simulink model "no_zerosimulink"  (R2017b)
settings: Solver=VariableStepAuto  StartTime=0.0  StopTime=10  RelTol=1e-3  EnableMultiTasking=on
undefined symbols (not defined in the file): DiscIntNeverNeededParam, rho1, rho3, rho5, rho6, sigma1, sigma2, sigma3, sigma4, sigma5, sigma6
libraries: simulink x1
settings Model: Creator=Tuo  LastModifiedBy=柏陞
settings OptimizationCC: LifeSpan=inf
settings DebuggingCC: SFUnexpectedBacktrackingDiag=warning  SFNoUnconditionalDefaultTransitionDiag=warning  SFExecutionAtInitializationDiag=none
settings CodeAppCC: StateflowObjectComments=on
settings GRTTargetCC: TargetLangStandard=C89/C90 (ANSI)  GeneratePreprocessorConditionals=Disable all
settings ConfigComp: CovMetricSettings=dw  CovHtmlReporting=on  CovSaveCumulativeToWorkspaceVar=on  CovSaveSingleToWorkspaceVar=on  CovExternalEMLEnable=off

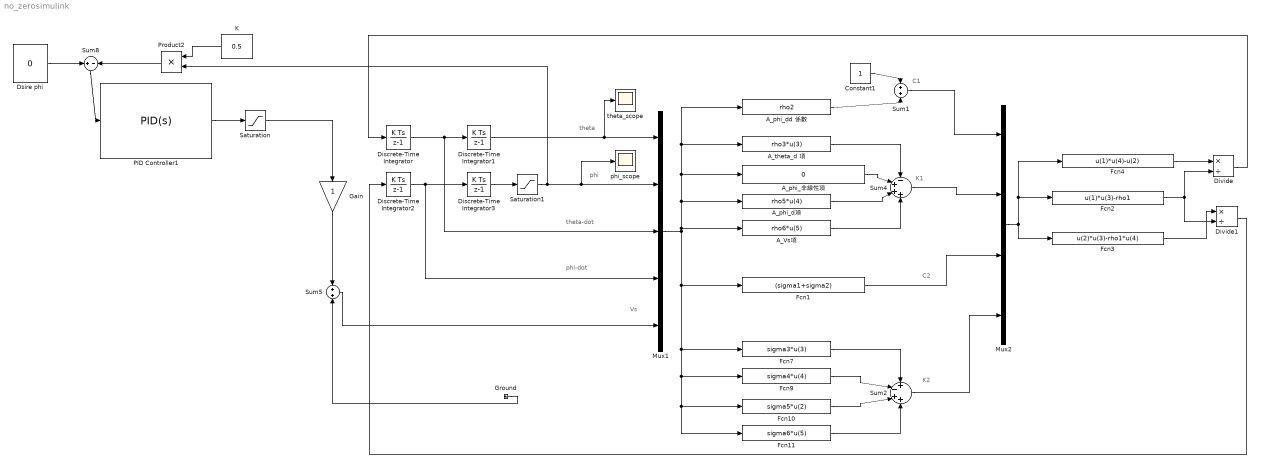
== system no_zerosimulink ==
  note: theta
  note: phi
  note: theta-dot
  note: phi-dot
  note: Vs
  note: K1
  note: C1
  note: K2
  note: C2
  A_Vs項 : Fcn  Expr=rho6*u(5)
  A_phi_dd 係數 : Fcn  Expr=rho2
  A_phi_d項 : Fcn  Expr=rho5*u(4)
  A_phi_非線性項 : Fcn  Expr=0
  A_theta_d 項 : Fcn  Expr=rho3*u(3)
  Constant1 : Constant  SampleTime=0.001
  Discrete-Time Integrator : DiscreteIntegrator  InitialConditionSetting=State (most efficient)  SampleTime=0.001  ICPrevOutput=DiscIntNeverNeededParam  ICPrevScaledInput=DiscIntNeverNeededParam
  Discrete-Time Integrator1 : DiscreteIntegrator  InitialConditionSetting=State (most efficient)  SampleTime=0.001  ICPrevOutput=DiscIntNeverNeededParam  ICPrevScaledInput=DiscIntNeverNeededParam
  Discrete-Time Integrator2 : DiscreteIntegrator  InitialConditionSetting=State (most efficient)  SampleTime=0.001  ICPrevOutput=DiscIntNeverNeededParam  ICPrevScaledInput=DiscIntNeverNeededParam
  Discrete-Time Integrator3 : DiscreteIntegrator  InitialCondition=pi/180  InitialConditionSetting=State (most efficient)  SampleTime=0.001  ICPrevOutput=DiscIntNeverNeededParam  ICPrevScaledInput=DiscIntNeverNeededParam
  Divide : Product  Inputs=*/
  Divide1 : Product  Inputs=*/
  Dsire phi : Constant  Value=0  SampleTime=0.001
  Fcn1 : Fcn  Expr=(sigma1+sigma2)
  Fcn10 : Fcn  Expr=sigma5*u(2)
  Fcn11 : Fcn  Expr=sigma6*u(5)
  Fcn2 : Fcn  Expr=u(1)*u(3)-rho1
  Fcn3 : Fcn  Expr=u(2)*u(3)-rho1*u(4)
  Fcn4 : Fcn  Expr=u(1)*u(4)-u(2)
  Fcn7 : Fcn  Expr=sigma3*u(3)
  Fcn9 : Fcn  Expr=sigma4*u(4)
  Gain : Gain
  Ground : Ground
  K : Constant  Value=0.5  SampleTime=0.001
  Mux1 : Mux  Inputs=5
  Mux2 : Mux
  PID Controller1 : simulink/Continuous/PID Controller  Controller=PID  TimeDomain=Continuous-time  SampleTime=-1  IntegratorMethod=Forward Euler  FilterMethod=Forward Euler  Form=Parallel  UseFilter=on  ControllerParametersSource=internal  P=0.02  I=0.06  D=0.0017  N=1000  InitialConditionSource=internal  InitialConditionForIntegrator=0  InitialConditionForFilter=0  ExternalReset=none  LimitOutput=off  UpperSaturationLimit=inf  LowerSaturationLimit=-inf  LinearizeAsGain=on  AntiWindupMode=none  Kb=1  TrackingMode=off  Kt=1  PParamMin=[]  PParamMax=[]  IParamMin=[]  IParamMax=[]  DParamMin=[]  DParamMax=[]  NParamMin=[]  NParamMax=[]  KbParamMin=[]  KbParamMax=[]  KtParamMin=[]  KtParamMax=[]  POutMin=[]  POutMax=[]  IOutMin=[]  IOutMax=[]  DOutMin=[]  DOutMax=[]  NOutMin=[]  NOutMax=[]  KbOutMin=[]  KbOutMax=[]  KtOutMin=[]  KtOutMax=[]  IntegratorOutMin=[]  IntegratorOutMax=[]  FilterOutMin=[]  FilterOutMax=[]  SumOutMin=[]  SumOutMax=[]  SumI1OutMin=[]  SumI1OutMax=[]  SumI2OutMin=[]  SumI2OutMax=[]  SumI3OutMin=[]  SumI3OutMax=[]  SumDOutMin=[]  SumDOutMax=[]  SaturationOutMin=[]  SaturationOutMax=[]  IntegratorContinuousStateAttributes=''  IntegratorStateMustResolveToSignalObject=off  IntegratorRTWStateStorageClass=Auto  FilterContinuousStateAttributes=''  FilterStateMustResolveToSignalObject=off  FilterRTWStateStorageClass=Auto  DifferentiatorICPrevScaledInput=0  DifferentiatorOutMin=[]  DifferentiatorOutMax=[]  InitialConditionSetting=State (most efficient)  FilterDiffOutCoefMin=[]  FilterDiffOutCoefMax=[]  SumDenOutMin=[]  SumDenOutMax=[]  SumNumOutMin=[]  SumNumOutMax=[]  ReciprocalOutMin=[]  ReciprocalOutMax=[]  DivideOutMin=[]  DivideOutMax=[]  TunerSelectOption=Transfer Function Based (PID Tuner App)
  Product2 : Product
  Saturation : Saturate  UpperLimit=255  LowerLimit=-255
  Saturation1 : Saturate  UpperLimit=1.57  LowerLimit=-1.57
  Sum1 : Sum
  Sum2 : Sum  Inputs=+-++
  Sum4 : Sum  Inputs=-+++
  Sum5 : Sum
  Sum8 : Sum  Inputs=+-
  phi_scope : Scope
  theta_scope : Scope
  wires:
  Discrete-Time Integrator/1 -> Mux1/3, Discrete-Time Integrator1/1
  Discrete-Time Integrator1/1 -> Mux1/1, theta_scope/1
  A_theta_d 項/1 -> Sum4/1
  A_phi_d項/1 -> Sum4/3
  A_Vs項/1 -> Sum4/4
  A_phi_dd 係數/1 -> Sum1/2
  Sum1/1 -> Mux2/1
  Constant1/1 -> Sum1/1
  Fcn7/1 -> Sum2/1
  Fcn9/1 -> Sum2/2
  Fcn10/1 -> Sum2/3
  Fcn11/1 -> Sum2/4
  Mux1/1 -> Fcn11/1, Fcn10/1, Fcn9/1, Fcn7/1, Fcn1/1, A_theta_d 項/1, A_phi_dd 係數/1, A_phi_非線性項/1, A_phi_d項/1, A_Vs項/1
  Sum4/1 -> Mux2/2
  Sum2/1 -> Mux2/4
  Mux2/1 -> Fcn4/1, Fcn2/1, Fcn3/1
  Divide/1 -> Discrete-Time Integrator/1
  Divide1/1 -> Discrete-Time Integrator2/1
  Discrete-Time Integrator2/1 -> Mux1/4, Discrete-Time Integrator3/1
  Discrete-Time Integrator3/1 -> Saturation1/1
  Saturation1/1 -> Mux1/2, phi_scope/1, Product2/2
  A_phi_非線性項/1 -> Sum4/2
  Fcn2/1 -> Divide/2, Divide1/2
  Fcn3/1 -> Divide1/1
  Fcn4/1 -> Divide/1
  Dsire phi/1 -> Sum8/1
  Product2/1 -> Sum8/2
  Sum8/1 -> PID Controller1/1
  K/1 -> Product2/1
  Fcn1/1 -> Mux2/3
  Sum5/1 -> Mux1/5
  Saturation/1 -> Gain/1
  Gain/1 -> Sum5/1
  Ground/1 -> Sum5/2
  PID Controller1/1 -> Saturation/1
